simulink model "followerAppl"  (R2022a)
settings: Solver=ode1  StartTime=0.0  StopTime=Inf  FixedStep=0.001  RelTol=1e-3
PostLoadFcn:
  | , if any(exist('dsrtsu_mdlpostloadfcn', 'file') ~= 0), dsrtsu_mdlpostloadfcn('Execute', bdroot); end,
  | 
  | % Begin Version: 1.0
  | if(3 == exist('DSWatchDog')), DSWatchDog('OpenModel', get_param(bdroot(gcs),'filename')); end; assignin('base', sprintf('DS_%s_STATE', upper(bdroot(gcs))), 0);
  | % End Version: 1.0
InitFcn:
  | , if any(exist('rtifpga_mdlclblib', 'file') ~= 0), rtifpga_mdlclblib('Init', bdroot); end,
  | , if any(exist('dsmpb_private', 'file') ~= 0), dsmpb_private('dsmpb_mdlclblib', 'Init', bdroot); end,
StartFcn:
  | % Begin Version: 1.0
  | if(3 == exist('DSWatchDog')), DSWatchDog('StartModel', get_param(bdroot(gcs),'filename')); end; assignin('base', sprintf('DS_%s_STATE', upper(bdroot(gcs))), 2);
  | % End Version: 1.0
StopFcn:
  | % Begin Version: 1.0
  | if(3 == exist('DSWatchDog')), DSWatchDog('StopModel', get_param(bdroot(gcs),'filename')); end; assignin('base', sprintf('DS_%s_STATE', upper(bdroot(gcs))), 0);
  | % End Version: 1.0
PreSaveFcn:
  | , if any(exist('dsmpb_private', 'file') ~= 0), dsmpb_private('dsmpb_mdlclblib', 'PreSave', bdroot); end,
  | 
  | % Begin Version: 1.0
  | OldName = get_param(bdroot(gcs), 'Tag'); NewName = get_param(bdroot(gcs), 'filename'); if (~strcmp(OldName, NewName)), if(3 == exist('DSWatchDog')), DSWatchDog('CloseModel', OldName); DSWatchDog('OpenModel', NewName); end; set_param(bdroot(gcs), 'Tag', NewName); end; try, evalin('base', 'clear OldName NewName'); catch, disp('Error during execution of PreSaveFcn callback'); end;
  | % End Version: 1.0
PostSaveFcn:
  | % Begin Version: 1.0
  | if(3 == exist('DSWatchDog')), DSWatchDog('SaveModel', get_param(bdroot(gcs),'filename')); end;
  | % End Version: 1.0
CloseFcn:
  | , if any(exist('dsmpb_private', 'file') ~= 0), dsmpb_private('dsmpb_mdlclblib', 'Close', bdroot); end,
  | % Begin Version: 1.0
  | if(3 == exist('DSWatchDog')), DSWatchDog('CloseModel', get_param(bdroot(gcs),'filename')); end; try, DS_STATE_NAME = sprintf('DS_%s_STATE', upper(bdroot(gcs))); evalin('base', 'clear(DS_STATE_NAME)'); evalin('base', 'clear DS_STATE_NAME'); catch, disp('Error during execution of CloseFcn callback'); end;
  | % End Version: 1.0
settings Model: Tag=C:\Users\dSPACE GmbH\Documents\dSPACE\Real-Time Testing\2023-B\SampleExperiments\TurnSignal_VEOSHYBRID\TurnSignal_VEOSHYBRID\Models\followerAppl.slx  RTICANMMDATA=struct('GeneralSetupData',struct('modelroot',['C:\Users\Admin\Documents\dSPACE\Real-Time Testing\2.6\SampleExperiments\TurnSignal_VEOSMC\Model'],'generalsettings',struct('filesettings',struct('destfolder',struct('Name','RTICANMM_FILES','Check',1),'buildfolder',struct('Name','.','Check',1),'AbsDestfolder',struct('Name',['C:\Users\Admin\Documents\dSPACE\Real-Time Testing\2.6\SampleExperiments\TurnSignal_VEOSMC\Model\RTICANMM_FILES']),'AbsBuildfolder',struct('Name',['C:\Users\Admin\Documents\dSPACE\Real-Time Testing\2.6\SampleExperiments\TurnSignal_VEOSMC\Model']))),'options',struct('addpaths',1,'rmpaths',1,'addtrcexclusion',logical(1),'cannavigator',struct('checkmonitoring',0),'show_usrtrc',0,'use_usrtrc',0),'advanced',struct('options',[1 1 1 1 1 1 1 1 1 1 1 1 1 1 1 1 1 1 1 1 1 1 1 1 1 1 1 1 1 1 1 1 1 1 1 1 1 1 1 1 1 1 1 1 1 1 1 1 1 1 1 1 1 1 1 1 1 1 1 1 1 1 1 1 1 1 1 1 1 1 1 1 1 1 1 1 1 1 1 1 1 1 1 1 1 1 1 1 1 1 1 1 1 1 1 1 1 1 1 1]),'MPSetup',{{}},'modelname','slaveAppl','block','slaveAppl'))  RTILINMMDATA=struct('GeneralSetupData',[])  DSRTSU_INTERNAL_RTI_VER=630  DSRTSU_INTERNAL_RTI_TYPE=rti1401  DSRTSU_INTERNAL_RTIFPGA=210  DSRTSU_INTERNAL_RTISTBM_VER=23.2  ModifiedByFormat=dSPACE GmbH  ExtModeTrigMode=oneshot  ExtModeArmWhenConnect=off  Creator=dSPACE GmbH  LastModifiedBy=dSPACE GmbH
settings SolverCC: AlgebraicLoopSolver=TrustRegion
settings DataIOCC: LimitDataPoints=on  SaveFormat=Structure  SignalLoggingSaveFormat=ModelDataLogs  ReturnWorkspaceOutputs=off
settings OptimizationCC: BlockReduction=off  ConditionallyExecuteInputs=off  OptimizeBlockIOStorage=off  BufferReuse=off  GlobalBufferReuse=off  ExpressionFolding=off  ExpressionDepthLimit=2147483647  LocalBlockOutputs=off  InitFltsAndDblsToZero=on  LifeSpan=inf
settings DebuggingCC: SaveWithParameterizedLinksMsg=none  UnderspecifiedInitializationDetection=Classic  MergeDetectMultiDrivingBlocksExec=none  SignalResolutionControl=TryResolveAllWithWarning  MultiTaskDSMMsg=warning  MultiTaskCondExecSysMsg=none  MultiTaskRateTransMsg=warning  TasksWithSamePriorityMsg=none  FcnCallInpInsideContextMsg=warning  UnconnectedInputMsg=warning  UnconnectedOutputMsg=warning  UnconnectedLineMsg=warning  StateNameClashWarn=warning  SFUnexpectedBacktrackingDiag=warning  SFNoUnconditionalDefaultTransitionDiag=warning  SFMachineParentedDataDiag=warning  ArithmeticOperatorsInVariantConditions=warning
settings HardwareCC: ProdBitPerLong=64  ProdLargestAtomicInteger=Integer  ProdWordSize=32  ProdHWDeviceType=Custom Processor->Custom  TargetIntDivRoundTo=Zero  TargetEndianess=LittleEndian  TargetHWDeviceType=Generic->Custom
settings ModelReferenceCC: PropagateSignalLabelsOutOfModel=off
settings SFSimCC: SimUseLocalCustomCode=off  CustomCodeUndefinedFunction=UseInterfaceOnly
settings RTWCC: Description=dSPACE Run-Time Target  SystemTargetFile=dsrt.tlc  GenCodeOnly=on  MakeCommand=make_dsrt  TemplateMakefile=dsrt_default_tmf  RTWVerbose=off  RTWUseLocalCustomCode=off
settings CodeAppCC: StateflowObjectComments=on
settings STFCustomTargetCC: ParMdlRefBuildCompliant=on  GRTInterface=off  SystemTargetFile=dsrt.tlc
settings GRTTargetCC: TargetLangStandard=C89/C90 (ANSI)  CompOptLevelCompliant=off  ConcurrentExecutionCompliant=off  CombineOutputUpdateFcns=off  MatFileLogging=off  CPPClassGenCompliant=off  UseToolchainInfoCompliant=off
settings ConfigComp: CovMetricSettings=dw  CovSaveCumulativeToWorkspaceVar=on  CovSaveSingleToWorkspaceVar=on  CovExternalEMLEnable=off  CovSFcnEnable=off

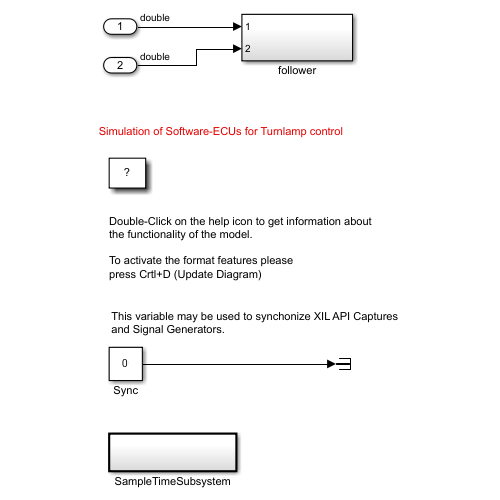
[thumbnail: Simulink's stored preview of the top-level diagram]
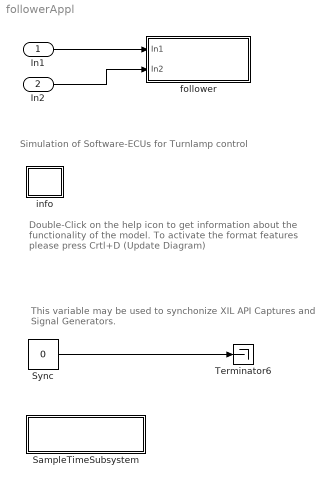
== system followerAppl ==
  note: Simulation of Software-ECUs for Turnlamp control
  note: Double-Click on the help icon to get information about
      | the functionality of the model.
      |
      | To activate the format features please
      | press Crtl+D (Update Diagram)
  note: This variable may be used to synchonize XIL API Captures
      | and Signal Generators.
  In1 : Inport  OutDataTypeStr=double  PortDimensions=1
  In2 : Inport  Port=2  OutDataTypeStr=double  PortDimensions=1
  SampleTimeSubsystem : Subsystem  TreatAsAtomicUnit=on  SystemSampleTime=0.01
  Sync : Constant  Value=0
  Terminator6 : Terminator
  follower : Subsystem
  info : Subsystem
      mask Display: disp('?')
  wires:
  In1/1 -> follower/1(In1)
  In2/1 -> follower/2(In2)
  Sync/1 -> Terminator6/1

== system followerAppl/SampleTimeSubsystem ==
  A1 : Constant  Value=0
  Terminator5 : Terminator
  info : Subsystem
      mask Display: disp('?')
  wires:
  A1/1 -> Terminator5/1

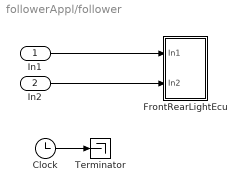
== system followerAppl/follower ==
  In1 : Inport
  In2 : Inport  Port=2
  Clock : Clock
  FrontRearLightEcu : Subsystem
  Terminator : Terminator
  wires:
  In1/1 -> FrontRearLightEcu/1(In1)
  In2/1 -> FrontRearLightEcu/2(In2)
  Clock/1 -> Terminator/1

== system followerAppl/info ==
  note: .
  note: This model simulates the behaviour of three ECUs for controlling TurnSignals,
      | dependent on a TurnSignalLever and a WarningLightSwitch
  note: Aim of this demo: to show possibilities of different ECU test procedures
  note: To control this model, use the corresponding ControlDesk experiment:
      | - Set TurnSignalLever to Left, Right or Off
      | - Switch WarningLight Switch to Off or On
      | - Change the Battery voltage: below a certain voltage level, some (simulated) malfunctions may occur
      |    - <= 7.2V, the ECUs will collapse completely
      |    - <= 8.2 V (dependent on voltage, more effect with lower voltage), simulated receiver in front and rear ECU become unstable,
      |      thus the timing of the generated TurnSignal will be disturbed

== system followerAppl/SampleTimeSubsystem/info ==
  note: .
  note: This subsystems realizes a new sampling period for measurements. It is configured with a step size of 10 ms.

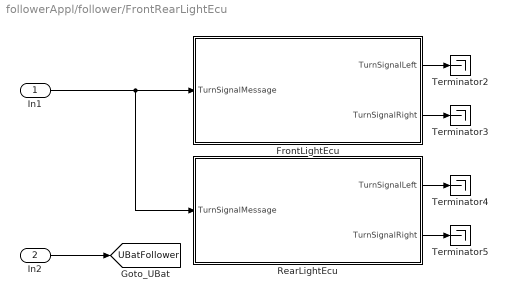
== system followerAppl/follower/FrontRearLightEcu ==
  In1 : Inport
  In2 : Inport  Port=2
  FrontLightEcu : Subsystem
  RearLightEcu : Subsystem
  Terminator{2..5} (4 alike) : Terminator
  tag scope: UBatFollower=global
  wires:
  In1/1 -> RearLightEcu/1(TurnSignalMessage), FrontLightEcu/1(TurnSignalMessage)
  FrontLightEcu/1(TurnSignalLeft) -> Terminator2/1
  FrontLightEcu/2(TurnSignalRight) -> Terminator3/1
  RearLightEcu/1(TurnSignalLeft) -> Terminator4/1
  RearLightEcu/2(TurnSignalRight) -> Terminator5/1
  In2/1 -> [UBatFollower]

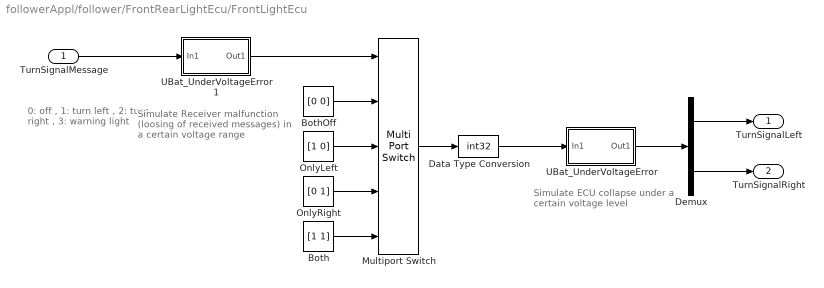
== system followerAppl/follower/FrontRearLightEcu/FrontLightEcu ==
  note: 0: off               ,
      | 1: turn left       ,
      | 2: turn right     ,
      | 3: warning light
  note: Simulate ECU collapse
      | under a certain voltage level
  note: Simulate Receiver malfunction
      | (loosing of received messages)
      | in a certain voltage range
  TurnSignalMessage : Inport
  Both : Constant  Value=[1 1]
  BothOff : Constant  Value=[0 0]
  Data Type Conversion : DataTypeConversion  OutDataTypeStr=int32  SaturateOnIntegerOverflow=off
  Demux : Demux  Outputs=2
  Multiport Switch : MultiPortSwitch  DataPortOrder=Zero-based contiguous  Inputs=4  zeroidx=on  SaturateOnIntegerOverflow=off  InputSameDT=off
  OnlyLeft : Constant  Value=[1 0]
  OnlyRight : Constant  Value=[0 1]
  UBat_UnderVoltageError : Subsystem
  UBat_UnderVoltageError1 : Subsystem
  TurnSignalLeft : Outport
  TurnSignalRight : Outport  Port=2
  wires:
  TurnSignalMessage/1 -> UBat_UnderVoltageError1/1(In1)
  BothOff/1 -> Multiport Switch/2
  OnlyLeft/1 -> Multiport Switch/3
  OnlyRight/1 -> Multiport Switch/4
  Both/1 -> Multiport Switch/5
  Multiport Switch/1 -> Data Type Conversion/1
  Data Type Conversion/1 -> UBat_UnderVoltageError/1(In1)
  UBat_UnderVoltageError/1(Out1) -> Demux/1
  Demux/1 -> TurnSignalLeft/1
  Demux/2 -> TurnSignalRight/1
  UBat_UnderVoltageError1/1(Out1) -> Multiport Switch/1

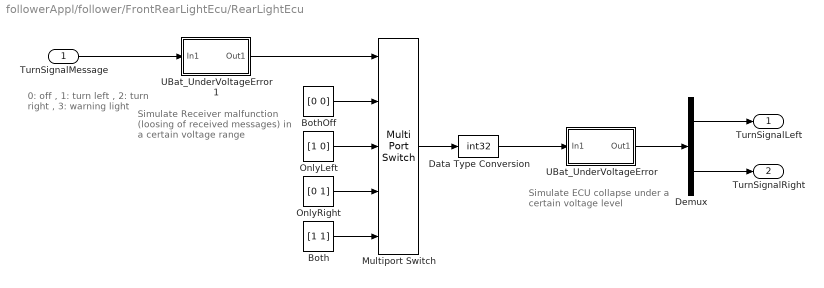
== system followerAppl/follower/FrontRearLightEcu/RearLightEcu ==
  note: 0: off               ,
      | 1: turn left       ,
      | 2: turn right     ,
      | 3: warning light
  note: Simulate Receiver malfunction
      | (loosing of received messages)
      | in a certain voltage range
  note: Simulate ECU collapse
      | under a certain voltage level
  TurnSignalMessage : Inport
  Both : Constant  Value=[1 1]
  BothOff : Constant  Value=[0 0]
  Data Type Conversion : DataTypeConversion  OutDataTypeStr=int32  SaturateOnIntegerOverflow=off
  Demux : Demux  Outputs=2
  Multiport Switch : MultiPortSwitch  DataPortOrder=Zero-based contiguous  Inputs=4  zeroidx=on  SaturateOnIntegerOverflow=off  InputSameDT=off
  OnlyLeft : Constant  Value=[1 0]
  OnlyRight : Constant  Value=[0 1]
  UBat_UnderVoltageError : Subsystem
  UBat_UnderVoltageError1 : Subsystem
  TurnSignalLeft : Outport
  TurnSignalRight : Outport  Port=2
  wires:
  UBat_UnderVoltageError1/1(Out1) -> Multiport Switch/1
  Demux/2 -> TurnSignalRight/1
  Demux/1 -> TurnSignalLeft/1
  UBat_UnderVoltageError/1(Out1) -> Demux/1
  Data Type Conversion/1 -> UBat_UnderVoltageError/1(In1)
  Multiport Switch/1 -> Data Type Conversion/1
  Both/1 -> Multiport Switch/5
  OnlyRight/1 -> Multiport Switch/4
  OnlyLeft/1 -> Multiport Switch/3
  BothOff/1 -> Multiport Switch/2
  TurnSignalMessage/1 -> UBat_UnderVoltageError1/1(In1)

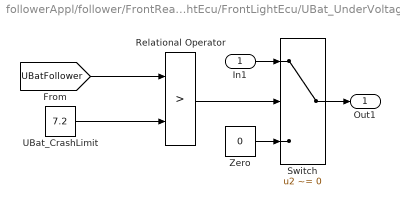
== system followerAppl/follower/FrontRearLightEcu/FrontLightEcu/UBat_UnderVoltageError ==
  In1 : Inport
  Relational Operator : RelationalOperator  Operator=>  OutDataTypeStr=boolean  InputSameDT=off
  Switch : Switch  Criteria=u2 ~= 0  SaturateOnIntegerOverflow=off  InputSameDT=off
  UBat_CrashLimit : Constant  Value=7.2
  Zero : Constant  Value=0
  Out1 : Outport
  wires:
  Switch/1 -> Out1/1
  In1/1 -> Switch/1
  Zero/1 -> Switch/3
  Relational Operator/1 -> Switch/2
  [UBatFollower] -> Relational Operator/1
  UBat_CrashLimit/1 -> Relational Operator/2

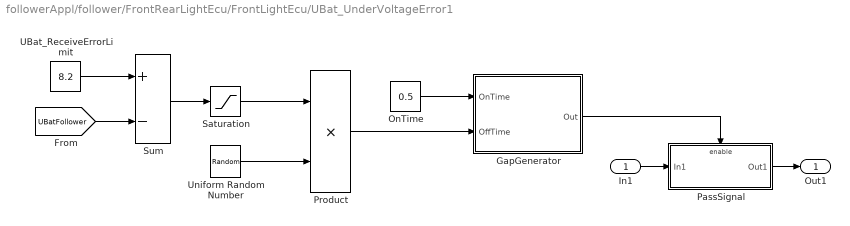
== system followerAppl/follower/FrontRearLightEcu/FrontLightEcu/UBat_UnderVoltageError1 ==
  In1 : Inport
  GapGenerator : Subsystem
  OnTime : Constant  Value=0.5
  PassSignal : Subsystem  TreatAsAtomicUnit=on
  Product : Product  RndMeth=Zero
  Saturation : Saturate  UpperLimit=1.2  LowerLimit=0.0
  Sum : Sum  Inputs=+-
  UBat_ReceiveErrorLimit : Constant  Value=8.2
  Uniform Random Number : UniformRandomNumber  Minimum=0  SampleTime=0
  Out1 : Outport
  wires:
  In1/1 -> PassSignal/1(In1)
  PassSignal/1(Out1) -> Out1/1
  GapGenerator/1(Out) -> PassSignal/Enable
  OnTime/1 -> GapGenerator/1(OnTime)
  Sum/1 -> Saturation/1
  UBat_ReceiveErrorLimit/1 -> Sum/1
  [UBatFollower] -> Sum/2
  Saturation/1 -> Product/1
  Product/1 -> GapGenerator/2(OffTime)
  Uniform Random Number/1 -> Product/2

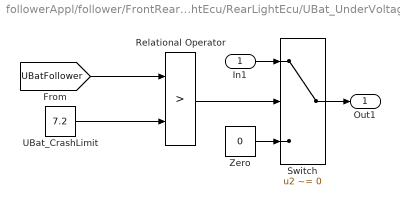
== system followerAppl/follower/FrontRearLightEcu/RearLightEcu/UBat_UnderVoltageError ==
  In1 : Inport
  Relational Operator : RelationalOperator  Operator=>  OutDataTypeStr=boolean  InputSameDT=off
  Switch : Switch  Criteria=u2 ~= 0  SaturateOnIntegerOverflow=off  InputSameDT=off
  UBat_CrashLimit : Constant  Value=7.2
  Zero : Constant  Value=0
  Out1 : Outport
  wires:
  UBat_CrashLimit/1 -> Relational Operator/2
  [UBatFollower] -> Relational Operator/1
  Relational Operator/1 -> Switch/2
  Zero/1 -> Switch/3
  In1/1 -> Switch/1
  Switch/1 -> Out1/1

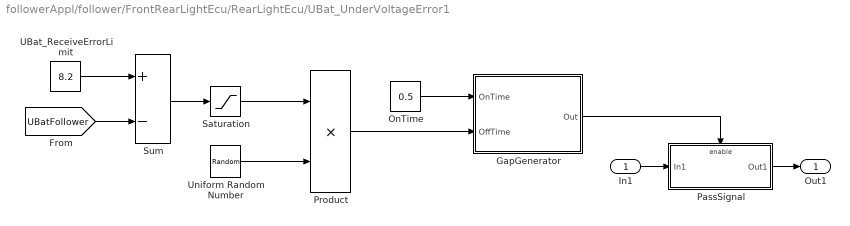
== system followerAppl/follower/FrontRearLightEcu/RearLightEcu/UBat_UnderVoltageError1 ==
  In1 : Inport
  GapGenerator : Subsystem
  OnTime : Constant  Value=0.5
  PassSignal : Subsystem  TreatAsAtomicUnit=on
  Product : Product  RndMeth=Zero
  Saturation : Saturate  UpperLimit=1.2  LowerLimit=0.0
  Sum : Sum  Inputs=+-
  UBat_ReceiveErrorLimit : Constant  Value=8.2
  Uniform Random Number : UniformRandomNumber  Minimum=0  Seed=1  SampleTime=0
  Out1 : Outport
  wires:
  Uniform Random Number/1 -> Product/2
  Product/1 -> GapGenerator/2(OffTime)
  Saturation/1 -> Product/1
  [UBatFollower] -> Sum/2
  UBat_ReceiveErrorLimit/1 -> Sum/1
  Sum/1 -> Saturation/1
  OnTime/1 -> GapGenerator/1(OnTime)
  GapGenerator/1(Out) -> PassSignal/Enable
  PassSignal/1(Out1) -> Out1/1
  In1/1 -> PassSignal/1(In1)

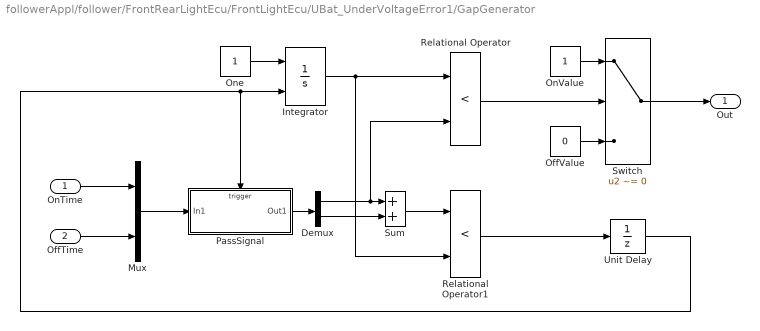
== system followerAppl/follower/FrontRearLightEcu/FrontLightEcu/UBat_UnderVoltageError1/GapGenerator ==
  OnTime : Inport
  OffTime : Inport  Port=2
  Demux : Demux  Outputs=2
  Integrator : Integrator  ExternalReset=rising
  Mux : Mux  Inputs=2
  OffValue : Constant  Value=0
  OnValue : Constant
  One : Constant
  PassSignal : Subsystem  TreatAsAtomicUnit=on
  Relational Operator : RelationalOperator  Operator=<  OutDataTypeStr=boolean  InputSameDT=off
  Relational Operator1 : RelationalOperator  Operator=<  OutDataTypeStr=boolean  InputSameDT=off
  Sum : Sum
  Switch : Switch  Criteria=u2 ~= 0  SaturateOnIntegerOverflow=off  InputSameDT=off
  Unit Delay : UnitDelay  InitialCondition=1  SampleTime=-1  HasFrameUpgradeWarning=on
  Out : Outport
  wires:
  Switch/1 -> Out/1
  Integrator/1 -> Relational Operator/1, Relational Operator1/2
  Relational Operator/1 -> Switch/2
  OnValue/1 -> Switch/1
  OffValue/1 -> Switch/3
  One/1 -> Integrator/1
  Sum/1 -> Relational Operator1/1
  Relational Operator1/1 -> Unit Delay/1
  Unit Delay/1 -> Integrator/2, PassSignal/Trigger
  Demux/1 -> Relational Operator/2, Sum/1
  Demux/2 -> Sum/2
  PassSignal/1(Out1) -> Demux/1
  Mux/1 -> PassSignal/1(In1)
  OnTime/1 -> Mux/1
  OffTime/1 -> Mux/2

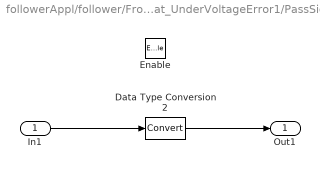
== system followerAppl/follower/FrontRearLightEcu/FrontLightEcu/UBat_UnderVoltageError1/PassSignal ==
  In1 : Inport
  Enable : EnablePort
  Data Type Conversion2 : DataTypeConversion  SaturateOnIntegerOverflow=off
  Out1 : Outport  InitialOutput=[0]
  wires:
  In1/1 -> Data Type Conversion2/1
  Data Type Conversion2/1 -> Out1/1

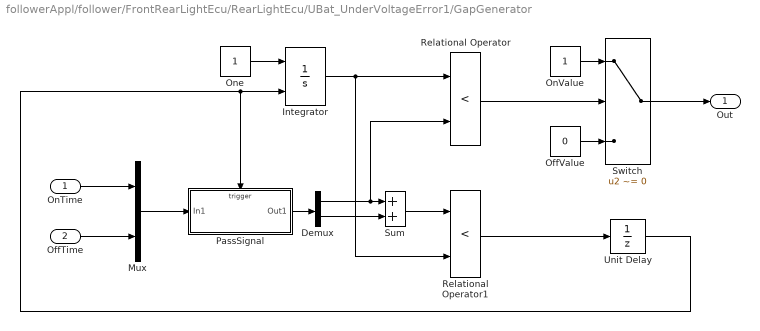
== system followerAppl/follower/FrontRearLightEcu/RearLightEcu/UBat_UnderVoltageError1/GapGenerator ==
  OnTime : Inport
  OffTime : Inport  Port=2
  Demux : Demux  Outputs=2
  Integrator : Integrator  ExternalReset=rising
  Mux : Mux  Inputs=2
  OffValue : Constant  Value=0
  OnValue : Constant
  One : Constant
  PassSignal : Subsystem  TreatAsAtomicUnit=on
  Relational Operator : RelationalOperator  Operator=<  OutDataTypeStr=boolean  InputSameDT=off
  Relational Operator1 : RelationalOperator  Operator=<  OutDataTypeStr=boolean  InputSameDT=off
  Sum : Sum
  Switch : Switch  Criteria=u2 ~= 0  SaturateOnIntegerOverflow=off  InputSameDT=off
  Unit Delay : UnitDelay  InitialCondition=1  SampleTime=-1  HasFrameUpgradeWarning=on
  Out : Outport
  wires:
  OffTime/1 -> Mux/2
  OnTime/1 -> Mux/1
  Mux/1 -> PassSignal/1(In1)
  PassSignal/1(Out1) -> Demux/1
  Demux/2 -> Sum/2
  Demux/1 -> Sum/1, Relational Operator/2
  Unit Delay/1 -> PassSignal/Trigger, Integrator/2
  Relational Operator1/1 -> Unit Delay/1
  Sum/1 -> Relational Operator1/1
  One/1 -> Integrator/1
  OffValue/1 -> Switch/3
  OnValue/1 -> Switch/1
  Relational Operator/1 -> Switch/2
  Integrator/1 -> Relational Operator1/2, Relational Operator/1
  Switch/1 -> Out/1

== system followerAppl/follower/FrontRearLightEcu/RearLightEcu/UBat_UnderVoltageError1/PassSignal ==
  In1 : Inport
  Enable : EnablePort
  Data Type Conversion2 : DataTypeConversion  SaturateOnIntegerOverflow=off
  Out1 : Outport  InitialOutput=[0]
  wires:
  Data Type Conversion2/1 -> Out1/1
  In1/1 -> Data Type Conversion2/1

== system followerAppl/follower/FrontRearLightEcu/FrontLightEcu/UBat_UnderVoltageError1/GapGenerator/PassSignal ==
  In1 : Inport
  Trigger : TriggerPort  VariantControl=Variant
  Gain : Gain
  Out1 : Outport  InitialOutput=[0.5 0]
  wires:
  In1/1 -> Gain/1
  Gain/1 -> Out1/1

== system followerAppl/follower/FrontRearLightEcu/RearLightEcu/UBat_UnderVoltageError1/GapGenerator/PassSignal ==
  In1 : Inport
  Trigger : TriggerPort  VariantControl=Variant
  Gain : Gain
  Out1 : Outport  InitialOutput=[0.5 0]
  wires:
  Gain/1 -> Out1/1
  In1/1 -> Gain/1
